simulink model "ZAD1_1_Model"  (R2018a)
settings: Solver=ode45  StartTime=0.0  StopTime=tend  MaxStep=Tp  RelTol=1e-3
values from neighbouring files (symbols this model uses):
  omega = 5.0    (= 5)    [ZAD1_Init.m]
  Qd1 = 0.2    [ZAD1_Init.m]
  Qd2 = 0.3    [ZAD1_Init.m]
  Qd3 = 0.4    [ZAD1_Init.m]
libraries: simulink x2
settings Model: Creator=szymon  LastModifiedBy=szymon

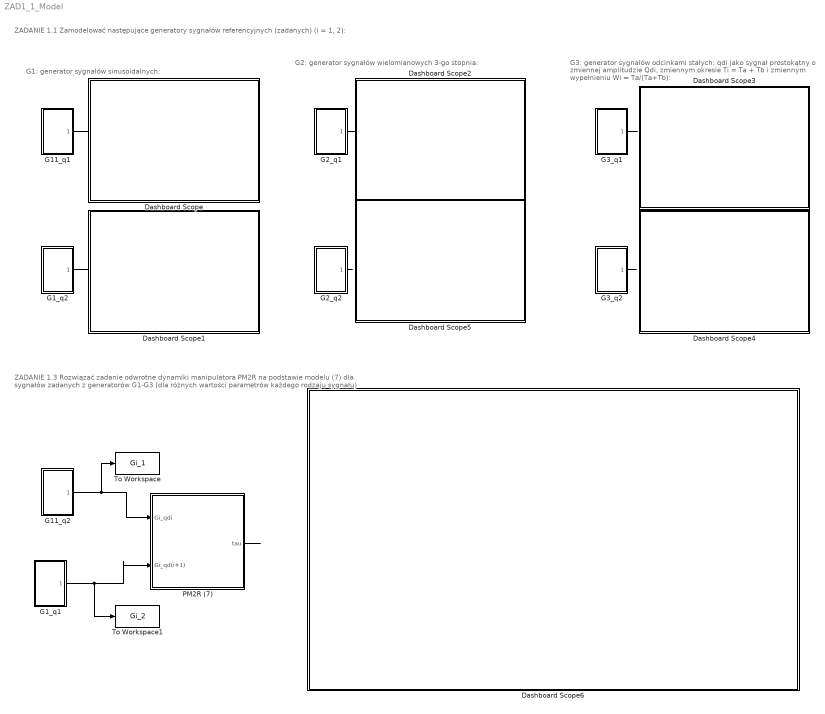
== system ZAD1_1_Model ==
  note: ZADANIE 1.1
      |  Zamodelować następujące generatory sygnałów referencyjnych (zadanych) (i = 1, 2):
  note: G1: generator sygnałów sinusoidalnych:
  note: G2: generator sygnałów wielomianowych 3-go stopnia:
  note: G3: generator sygnałów odcinkami stałych: qdi jako sygnał
      | prostokątny o zmiennej amplitudzie Qdi, zmiennym okresie
      | Ti = Ta + Tb i zmiennym wypełnieniu Wi = Ta/(Ta+Tb):
  note: ZADANIE 1.3
      | Rozwiązać zadanie odwrotne dynamiki manipulatora PM2R na podstawie modelu (7) dla sygnałów zadanych z generatorów G1-G3 (dla różnych wartości parametrów każdego rodzaju sygnału)
  Dashboard Scope : Subsystem  DialogController=hmiCreateDDGDialog  IsWebBlock=on  mask(MWDashboardBlock){webBlockId=04488d21-9573-4550-ab8f-f6209d6c8a1b, webBlockType=sdiscope, ShowInitialText=on, HMISrcModelName=ZAD1_1_Model}
      mask prompts: webBlockId "WebBlock Id"; webBlockType "WebBlock Type"; HMISrcModelName "Source Model"
      mask help: SimulinkHMI:dialogs:HMIScopeDialogDesc
      mask Help: helpview([docroot '/mapfiles/simulink.map'], 'hmi_scope')
      mask Display:
      | if strcmp(get_param(bdroot(gcb),'BlockDiagramType'), 'library')
      |     image([(matlabroot) '/toolbox/simulink/hmi/icons/DashboardScope.png']);
      | end
  Dashboard Scope1 : Subsystem  DialogController=hmiCreateDDGDialog  IsWebBlock=on  mask(MWDashboardBlock){webBlockId=237970db-90af-416d-bf1d-dfbb7f9e9cad, webBlockType=sdiscope, ShowInitialText=on, HMISrcModelName=ZAD1_1_Model}
      mask prompts: webBlockId "WebBlock Id"; webBlockType "WebBlock Type"; HMISrcModelName "Source Model"
      mask help: SimulinkHMI:dialogs:HMIScopeDialogDesc
      mask Help: helpview([docroot '/mapfiles/simulink.map'], 'hmi_scope')
      mask Display:
      | if strcmp(get_param(bdroot(gcb),'BlockDiagramType'), 'library')
      |     image([(matlabroot) '/toolbox/simulink/hmi/icons/DashboardScope.png']);
      | end
  Dashboard Scope2 : Subsystem  DialogController=hmiCreateDDGDialog  IsWebBlock=on  mask(MWDashboardBlock){webBlockId=b7179730-6836-4ef5-be25-0ee232a07c3f, webBlockType=sdiscope, ShowInitialText=on, HMISrcModelName=ZAD1_1_Model}
      mask prompts: webBlockId "WebBlock Id"; webBlockType "WebBlock Type"; HMISrcModelName "Source Model"
      mask help: SimulinkHMI:dialogs:HMIScopeDialogDesc
      mask Help: helpview([docroot '/mapfiles/simulink.map'], 'hmi_scope')
      mask Display:
      | if strcmp(get_param(bdroot(gcb),'BlockDiagramType'), 'library')
      |     image([(matlabroot) '/toolbox/simulink/hmi/icons/DashboardScope.png']);
      | end
  Dashboard Scope3 : Subsystem  DialogController=hmiCreateDDGDialog  IsWebBlock=on  mask(MWDashboardBlock){webBlockId=3d08afb7-3216-472b-a002-dff68bb25804, webBlockType=sdiscope, ShowInitialText=on, HMISrcModelName=ZAD1_1_Model}
      mask prompts: webBlockId "WebBlock Id"; webBlockType "WebBlock Type"; HMISrcModelName "Source Model"
      mask help: SimulinkHMI:dialogs:HMIScopeDialogDesc
      mask Help: helpview([docroot '/mapfiles/simulink.map'], 'hmi_scope')
      mask Display:
      | if strcmp(get_param(bdroot(gcb),'BlockDiagramType'), 'library')
      |     image([(matlabroot) '/toolbox/simulink/hmi/icons/DashboardScope.png']);
      | end
  Dashboard Scope4 : Subsystem  DialogController=hmiCreateDDGDialog  IsWebBlock=on  mask(MWDashboardBlock){webBlockId=5c56396f-8b35-4fe7-82c8-f069b0160f5a, webBlockType=sdiscope, ShowInitialText=on, HMISrcModelName=ZAD1_1_Model}
      mask prompts: webBlockId "WebBlock Id"; webBlockType "WebBlock Type"; HMISrcModelName "Source Model"
      mask help: SimulinkHMI:dialogs:HMIScopeDialogDesc
      mask Help: helpview([docroot '/mapfiles/simulink.map'], 'hmi_scope')
      mask Display:
      | if strcmp(get_param(bdroot(gcb),'BlockDiagramType'), 'library')
      |     image([(matlabroot) '/toolbox/simulink/hmi/icons/DashboardScope.png']);
      | end
  Dashboard Scope5 : Subsystem  DialogController=hmiCreateDDGDialog  IsWebBlock=on  mask(MWDashboardBlock){webBlockId=43fb1c02-49ac-48a2-8cec-79fa1d2745da, webBlockType=sdiscope, ShowInitialText=on, HMISrcModelName=ZAD1_1_Model}
      mask prompts: webBlockId "WebBlock Id"; webBlockType "WebBlock Type"; HMISrcModelName "Source Model"
      mask help: SimulinkHMI:dialogs:HMIScopeDialogDesc
      mask Help: helpview([docroot '/mapfiles/simulink.map'], 'hmi_scope')
      mask Display:
      | if strcmp(get_param(bdroot(gcb),'BlockDiagramType'), 'library')
      |     image([(matlabroot) '/toolbox/simulink/hmi/icons/DashboardScope.png']);
      | end
  Dashboard Scope6 : Subsystem  DialogController=hmiCreateDDGDialog  IsWebBlock=on  mask(MWDashboardBlock){webBlockId=060137c1-44cd-42f9-89eb-7b1da18c6d2d, webBlockType=sdiscope, ShowInitialText=on, HMISrcModelName=ZAD1_1_Model}
      mask prompts: webBlockId "WebBlock Id"; webBlockType "WebBlock Type"; HMISrcModelName "Source Model"
      mask help: SimulinkHMI:dialogs:HMIScopeDialogDesc
      mask Help: helpview([docroot '/mapfiles/simulink.map'], 'hmi_scope')
      mask Display:
      | if strcmp(get_param(bdroot(gcb),'BlockDiagramType'), 'library')
      |     image([(matlabroot) '/toolbox/simulink/hmi/icons/DashboardScope.png']);
      | end
  G11_q1 : Subsystem
  G11_q2 : Subsystem
  G1_q1 : Subsystem
  G1_q2 : Subsystem
  G2_q1 : Subsystem
  G2_q2 : Subsystem
  G3_q1 : Subsystem
  G3_q2 : Subsystem
  PM2R (7) : Subsystem
  To Workspace : ToWorkspace  VariableName=Gi_1  SampleTime=-1
  To Workspace1 : ToWorkspace  VariableName=Gi_2  SampleTime=-1
  wires:
  G11_q1/1(G1_q1) -> ?
  G1_q2/1(G1_q2) -> ?
  G2_q1/1(G2_q1) -> ?
  G3_q2/1(G3_q2) -> ?
  G3_q1/1(G3_q1) -> ?
  G2_q2/1(G2_q1) -> ?
  G11_q2/1(G1_q1) -> To Workspace/1, PM2R (7)/1(Gi_qdi)
  G1_q1/1(G1_q2) -> To Workspace1/1, PM2R (7)/2(Gi_qd(i+1))
  PM2R (7)/1(tau) -> ?

== system ZAD1_1_Model/Dashboard Scope ==

== system ZAD1_1_Model/Dashboard Scope1 ==

== system ZAD1_1_Model/Dashboard Scope2 ==

== system ZAD1_1_Model/Dashboard Scope3 ==

== system ZAD1_1_Model/Dashboard Scope4 ==

== system ZAD1_1_Model/Dashboard Scope5 ==

== system ZAD1_1_Model/Dashboard Scope6 ==

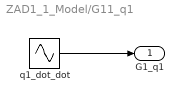
== system ZAD1_1_Model/G11_q1 ==
  "q1_dot_dot " : Sin  Amplitude=-omega^2*Qd1  SampleTime=0
  G1_q1 : Outport
  wires:
  "q1_dot_dot "/1 -> G1_q1/1

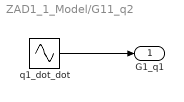
== system ZAD1_1_Model/G11_q2 ==
  "q1_dot_dot " : Sin  Amplitude=-omega^2*Qd1  SampleTime=0
  G1_q1 : Outport
  wires:
  "q1_dot_dot "/1 -> G1_q1/1

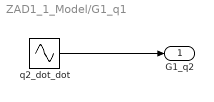
== system ZAD1_1_Model/G1_q1 ==
  "q2_dot_dot " : Sin  Amplitude=-omega^2*Qd2  SampleTime=0
  G1_q2 : Outport
  wires:
  "q2_dot_dot "/1 -> G1_q2/1

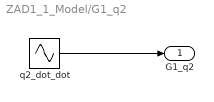
== system ZAD1_1_Model/G1_q2 ==
  "q2_dot_dot " : Sin  Amplitude=-omega^2*Qd2  SampleTime=0
  G1_q2 : Outport
  wires:
  "q2_dot_dot "/1 -> G1_q2/1

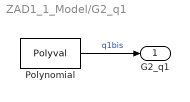
== system ZAD1_1_Model/G2_q1 ==
  Polynomial : Polyval  Coefs=[6*Qd3*t, 2*Qd2]
  G2_q1 : Outport
  wires:
  Polynomial/1 -> G2_q1/1  "q1bis"

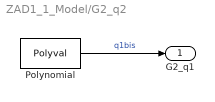
== system ZAD1_1_Model/G2_q2 ==
  Polynomial : Polyval  Coefs=[6*Qd2*t, 2*Qd1]
  G2_q1 : Outport
  wires:
  Polynomial/1 -> G2_q1/1  "q1bis"

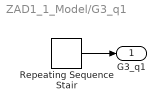
== system ZAD1_1_Model/G3_q1 ==
  Repeating Sequence Stair : simulink/Sources/Repeating Sequence Stair  OutValues=[Qd1 -Qd1 -Qd1].'  tsamp=Ta  OutMin=[]  OutMax=[]  OutDataTypeStr=double  OutputDataTypeScalingMode=double  OutDataType=fixdt(0,8)  ConRadixGroup=Best Precision: Vector-wise  OutScaling=2^-12
  G3_q1 : Outport
  wires:
  Repeating Sequence Stair/1 -> G3_q1/1

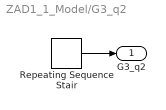
== system ZAD1_1_Model/G3_q2 ==
  Repeating Sequence Stair : simulink/Sources/Repeating Sequence Stair  OutValues=[Qd2 -Qd2 -Qd2].'  tsamp=Ta  OutMin=[]  OutMax=[]  OutDataTypeStr=double  OutputDataTypeScalingMode=double  OutDataType=fixdt(0,8)  ConRadixGroup=Best Precision: Vector-wise  OutScaling=2^-12
  G3_q2 : Outport
  wires:
  Repeating Sequence Stair/1 -> G3_q2/1

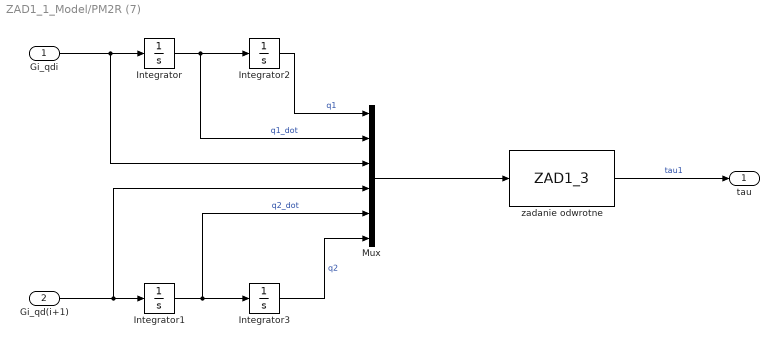
== system ZAD1_1_Model/PM2R (7) ==
  Gi_qdi : Inport
  Gi_qd(i+1) : Inport  Port=2
  Integrator{,1..3} (4 alike) : Integrator
  Mux : Mux  Inputs=6
  zadanie odwrotne : MATLABFcn  MATLABFcn=ZAD1_3
  tau : Outport
  wires:
  Integrator/1 -> Mux/2, Integrator2/1  "q1_dot"
  Integrator1/1 -> Mux/5, Integrator3/1  "q2_dot"
  Gi_qdi/1 -> Mux/3, Integrator/1
  Integrator3/1 -> Mux/6  "q2"
  Gi_qd(i+1)/1 -> Mux/4, Integrator1/1
  Integrator2/1 -> Mux/1  "q1"
  Mux/1 -> zadanie odwrotne/1
  zadanie odwrotne/1 -> tau/1  "tau1"
